simulink model "SPMe_EqCM"  (R2024a)
settings: Solver=FixedStepAuto  StartTime=0.0  StopTime=t_end  FixedStep=dt  MaxStep=1  RelTol=1e-6
values from neighbouring files (symbols this model uses):
  alpha = 64.526    [EqCM.m]
  dt = 0.2    [run_SPMe_fast_discharge.m]    (also in run_SPMe_sweep.m = param.dt; run_SPMe_vent.m = param.dt)
  I = 4.6*C_rates(c)    [run_SPMe_fast_discharge.m]    (also in run_SPMe_sweep.m; run_SPMe_vent.m = squeeze(sol.I.Data))
  p0 = [0.114319142120841  -0.663997904709863          1.686768366470837  -2.462409468590447   2.282769243949050          -1.401600551327618   0.576551904459066  -0.157044814050174          0.027351974716897  -0.002866912229499   0.000171009483610         0.000029999998915].*1e5    [run_SPMe_vent.m]
  Q_nom = 4.6    [run_SPMe_fast_discharge.m]    (also in run_SPMe_sweep.m; run_SPMe_vent.m)
  Rs = [0.051109270053841  -0.124390708105661             0.112323360710586  -0.046901650715843 0.015533047683140]             *z.^(4:-1:0)'    [EqCM.m]
  T_amb = 273.15+25    (= 298.15)    [EqCM.m]    (also in run_SPMe_vent.m = param.T_amb)
  V_min = 0    [run_SPMe_fast_discharge.m]    (also in run_SPMe_sweep.m; run_SPMe_vent.m = -3)
undefined symbols (not defined in the file or in its folder): A, DMC, E_p, EC, L_p0, m_an, M_C6, P_atm, P_crit, R, R_tab, sigma_0, SOC_0, V_head_0, x0, x_sei_0, y_dmc, y_ec
libraries: simulink x1
settings Model: Creator=tom  LastModifiedBy=Vivian
settings SolverCC: AlgebraicLoopSolver=TrustRegion
settings DebuggingCC: UnconnectedInputMsg=warning  UnconnectedOutputMsg=warning  UnconnectedLineMsg=warning
settings ModelReferenceCC: EnableRefExpFcnMdlSchedulingChecks=on
settings RTWCC: GPUComputeCapability=3.5  DLArmComputeVersion=19.05

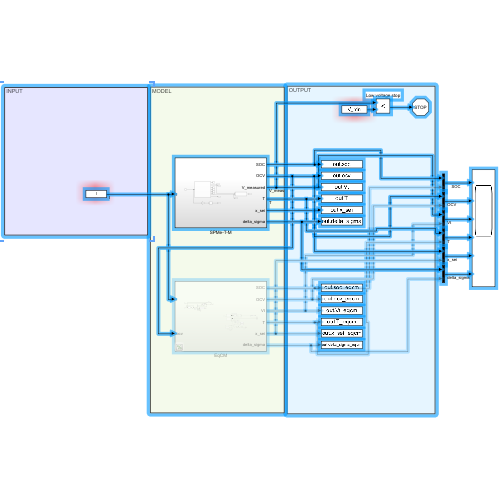
[thumbnail: Simulink's stored preview of the top-level diagram]
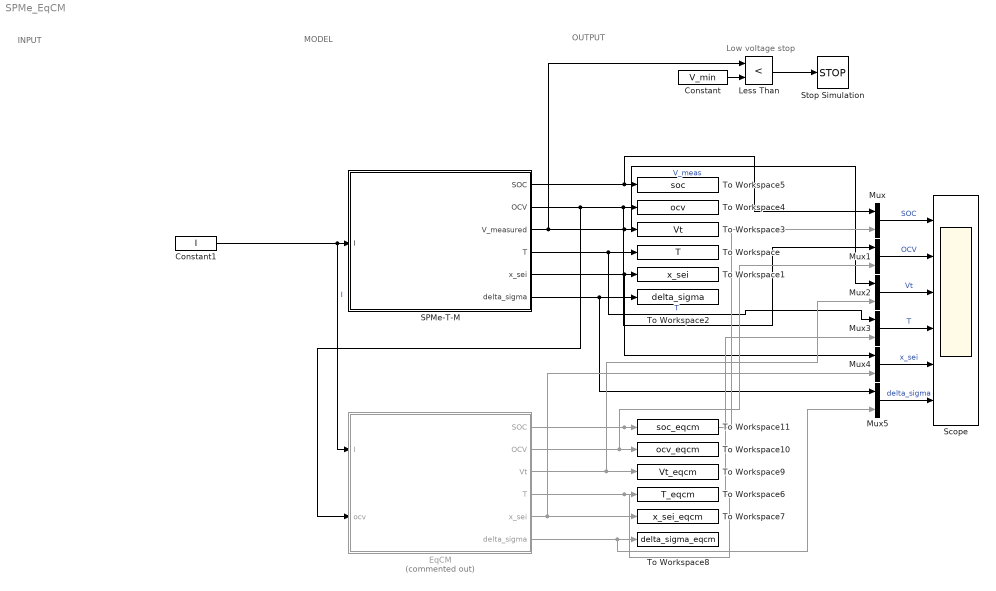
== system SPMe_EqCM ==
  note: OUTPUT
  note: MODEL
  note: INPUT
  note: Low voltage stop
  Constant : Constant  Value=V_min
  Constant1 : Constant  Value=I
  EqCM : Subsystem  Commented=on
  Less Than : RelationalOperator  Operator=<  OutDataTypeStr=boolean  RndMeth=Simplest  InputSameDT=off
  Mux{,1..5} (6 alike) : Mux  Inputs=2
  SPMe-T-M : Subsystem
  Scope : Scope  NumInputPorts=6
  Stop Simulation : Stop
  To Workspace : ToWorkspace  VariableName=T  SaveFormat=Timeseries  SampleTime=-1
  To Workspace1 : ToWorkspace  VariableName=x_sei  SaveFormat=Timeseries  SampleTime=-1
  To Workspace10 : ToWorkspace  VariableName=ocv_eqcm  SaveFormat=Timeseries  SampleTime=-1
  To Workspace11 : ToWorkspace  VariableName=soc_eqcm  SaveFormat=Timeseries  SampleTime=-1
  To Workspace2 : ToWorkspace  VariableName=delta_sigma  SaveFormat=Timeseries  SampleTime=-1
  To Workspace3 : ToWorkspace  VariableName=Vt  SaveFormat=Timeseries  SampleTime=-1
  To Workspace4 : ToWorkspace  VariableName=ocv  SaveFormat=Timeseries  SampleTime=-1
  To Workspace5 : ToWorkspace  VariableName=soc  SaveFormat=Timeseries  SampleTime=-1
  To Workspace6 : ToWorkspace  VariableName=T_eqcm  SaveFormat=Timeseries  SampleTime=-1
  To Workspace7 : ToWorkspace  VariableName=x_sei_eqcm  SaveFormat=Timeseries  SampleTime=-1
  To Workspace8 : ToWorkspace  VariableName=delta_sigma_eqcm  SaveFormat=Timeseries  SampleTime=-1
  To Workspace9 : ToWorkspace  VariableName=Vt_eqcm  SaveFormat=Timeseries  SampleTime=-1
  wires:
  Less Than/1 -> Stop Simulation/1
  Constant/1 -> Less Than/2
  SPMe-T-M/3(V_measured) -> Mux2/1, To Workspace3/1, Less Than/1  "V_meas"
  Constant1/1 -> EqCM/1(I), SPMe-T-M/1(I)  "I"
  SPMe-T-M/4(T) -> Mux3/1, To Workspace/1  "T"
  SPMe-T-M/5(x_sei) -> Mux4/1, To Workspace1/1
  SPMe-T-M/6(delta_sigma) -> Mux5/1, To Workspace2/1
  SPMe-T-M/2(OCV) -> EqCM/2(ocv), Mux1/1, To Workspace4/1
  SPMe-T-M/1(SOC) -> Mux/1, To Workspace5/1
  EqCM/1(SOC) -> Mux/2, To Workspace11/1
  EqCM/2(OCV) -> Mux1/2, To Workspace10/1
  EqCM/3(Vt) -> Mux2/2, To Workspace9/1
  EqCM/4(T) -> Mux3/2, To Workspace6/1
  Mux/1 -> Scope/1  "SOC"
  Mux1/1 -> Scope/2  "OCV"
  Mux2/1 -> Scope/3  "Vt"
  Mux3/1 -> Scope/4  "T"
  Mux4/1 -> Scope/5  "x_sei"
  Mux5/1 -> Scope/6  "delta_sigma"
  EqCM/5(x_sei) -> Mux4/2, To Workspace7/1
  EqCM/6(delta_sigma) -> Mux5/2, To Workspace8/1

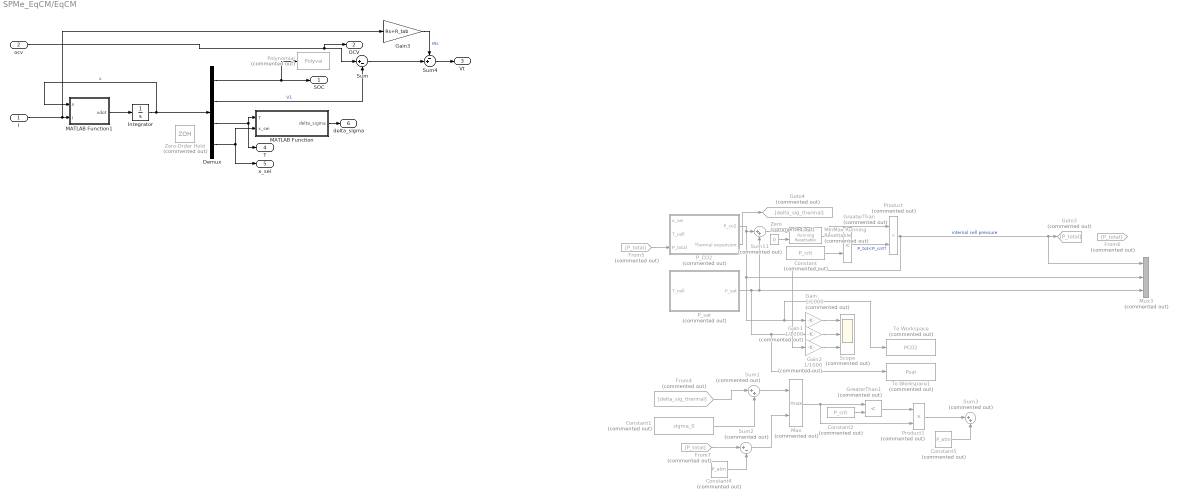
== system SPMe_EqCM/EqCM ==
  I : Inport
  ocv : Inport  Port=2
  Constant : Constant  Commented=on  Value=P_crit
  Constant1 : Constant  Commented=on  Value=sigma_0
  Constant2 : Constant  Commented=on  Value=P_crit
  Constant4 : Constant  Commented=on  Value=P_atm
  Constant5 : Constant  Commented=on  Value=P_atm
  Demux : Demux
  From4 : From  Commented=on  GotoTag=delta_sig_thermal
  From5 : From  Commented=on  GotoTag=P_total
  From6 : From  Commented=on  GotoTag=P_total
  From7 : From  Commented=on  GotoTag=P_total
  Gain : Gain  Commented=on  Gain=1/1000
  Gain1 : Gain  Commented=on  Gain=1/1000
  Gain2 : Gain  Commented=on  Gain=1/1000
  Gain3 : Gain  Gain=Rs+R_tab
  Goto3 : Goto  Commented=on  GotoTag=P_total
  Goto4 : Goto  Commented=on  GotoTag=delta_sig_thermal
  GreaterThan : RelationalOperator  Commented=on  Operator=<  OutDataTypeStr=boolean  RndMeth=Simplest  InputSameDT=off
  GreaterThan1 : RelationalOperator  Commented=on  Operator=<  OutDataTypeStr=boolean  RndMeth=Simplest  InputSameDT=off
  Integrator : Integrator  InitialCondition=x0'
  MATLAB Function : MATLAB Function  TreatAsAtomicUnit=on
  MATLAB Function1 : MATLAB Function  TreatAsAtomicUnit=on
  Max : MinMax  Commented=on  Function=max  Inputs=2
  MinMax Running Resettable : simulink/Math Operations/MinMax Running Resettable  Commented=on  Function=max  vinit=0
  Mux3 : Mux  Commented=on  Inputs=3
  P_CO2 : Subsystem  Commented=on
  P_sat : Subsystem  Commented=on
  Polynomial : Polyval  Commented=on  Coefs=p0
  Product : Product  Commented=on
  Product1 : Product  Commented=on
  Scope : Scope  Commented=on  NumInputPorts=3
  Sum : Sum  Inputs=|+-
  Sum1 : Sum  Commented=on  Inputs=|++
  Sum11 : Sum  Commented=on  Inputs=|++
  Sum2 : Sum  Commented=on  Inputs=|+-
  Sum3 : Sum  Commented=on  Inputs=|++
  Sum4 : Sum  Inputs=-+|
  To Workspace : ToWorkspace  Commented=on  VariableName=PCO2  SaveFormat=Timeseries  SampleTime=-1
  To Workspace1 : ToWorkspace  Commented=on  VariableName=Psat  SaveFormat=Timeseries  SampleTime=-1
  Zero : Constant  Commented=on  Value=0  OutDataTypeStr=Inherit: Inherit via back propagation
  Zero-Order Hold : ZeroOrderHold  Commented=on  SampleTime=dt
  SOC : Outport
  OCV : Outport  Port=2
  Vt : Outport  Port=3
  T : Outport  Port=4
  x_sei : Outport  Port=5
  delta_sigma : Outport  Port=6
  wires:
  I/1 -> Gain3/1, MATLAB Function1/2(I)
  From7/1 -> Sum2/1
  Sum11/1 -> MinMax Running Resettable/1
  Zero/1 -> MinMax Running Resettable/2
  GreaterThan/1 -> Product/2  "P_tot<P_crit?"
  Gain2/1 -> Scope/3
  Constant1/1 -> Sum1/2
  Constant4/1 -> Sum2/2
  Constant/1 -> GreaterThan/2
  Sum1/1 -> Max/1
  Constant2/1 -> GreaterThan1/2
  P_sat/1(P_sat) -> To Workspace1/1, Gain1/1, Sum11/2, Mux3/3
  Constant5/1 -> Sum3/2
  MinMax Running Resettable/1 -> Product/1, GreaterThan/1
  Product1/1 -> Sum3/1
  From4/1 -> Sum1/1
  Gain/1 -> Scope/1
  From5/1 -> P_CO2/3(P_total)
  Product/1 -> Gain2/1, Mux3/1, Goto3/1  "internal cell pressure"
  Max/1 -> GreaterThan1/1, Product1/2
  Gain1/1 -> Scope/2
  GreaterThan1/1 -> Product1/1
  P_CO2/1(P_co2) -> To Workspace/1, Gain/1, Mux3/2, Sum11/1
  P_CO2/2(Thermal expansion) -> Goto4/1
  Sum2/1 -> Max/2
  MATLAB Function/1(delta_sigma) -> delta_sigma/1
  MATLAB Function1/1(xdot) -> Integrator/1
  Integrator/1 -> Demux/1, MATLAB Function1/1(x)  "x"
  Demux/3 -> T/1, MATLAB Function/1(T)
  Demux/4 -> x_sei/1, MATLAB Function/2(x_sei)
  Demux/1 -> Polynomial/1, SOC/1
  Demux/2 -> Sum/2  "V1"
  Gain3/1 -> Sum4/1  "IRs"
  Sum/1 -> Sum4/2
  Sum4/1 -> Vt/1
  ocv/1 -> OCV/1, Sum/1

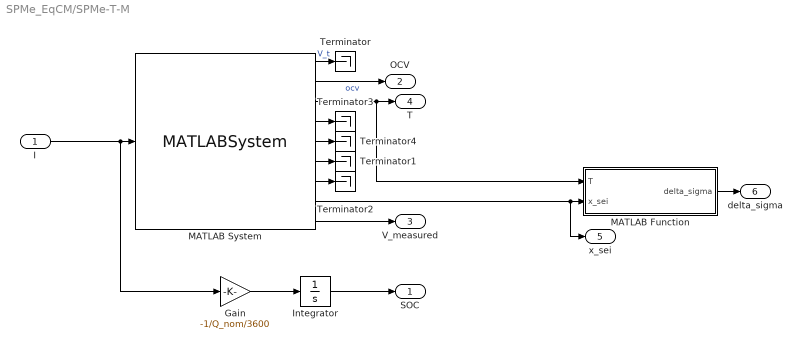
== system SPMe_EqCM/SPMe-T-M ==
  I : Inport
  Gain : Gain  Gain=-1/Q_nom/3600
  Integrator : Integrator  InitialCondition=SOC_0
  MATLAB Function : MATLAB Function  TreatAsAtomicUnit=on
  MATLAB System : MATLABSystem  System=pybamm_bat  SimulateUsing=Interpreted execution
      mask Type: pybamm_bat
      mask Display:
      | disp('pybamm_bat');
      | port_label('input',1,'current');
      | port_label('output',1,'V_t');
      | port_label('output',2,'ocv');
      | port_label('output',3,'T');
      | port_label('output',4,'ce');
      | port_label('output',5,'heating');
      | port_label('output',6,'neg_conc');
      | port_label('output',7,'pos_conc');
      | port_label('output',8,'x_sei');
      | port_label('output',9,'V_meas');
  Terminator{,1..4} (5 alike) : Terminator
  SOC : Outport
  OCV : Outport  Port=2
  V_measured : Outport  Port=3
  T : Outport  Port=4
  x_sei : Outport  Port=5
  delta_sigma : Outport  Port=6
  wires:
  MATLAB System/9 -> V_measured/1
  MATLAB System/3 -> MATLAB Function/1(T), T/1
  MATLAB System/8 -> x_sei/1, MATLAB Function/2(x_sei)
  MATLAB Function/1(delta_sigma) -> delta_sigma/1
  MATLAB System/1 -> Terminator/1  "V_t"
  MATLAB System/6 -> Terminator1/1
  MATLAB System/7 -> Terminator2/1
  MATLAB System/4 -> Terminator3/1
  MATLAB System/5 -> Terminator4/1
  MATLAB System/2 -> OCV/1  "ocv"
  I/1 -> Gain/1, MATLAB System/1
  Integrator/1 -> SOC/1
  Gain/1 -> Integrator/1

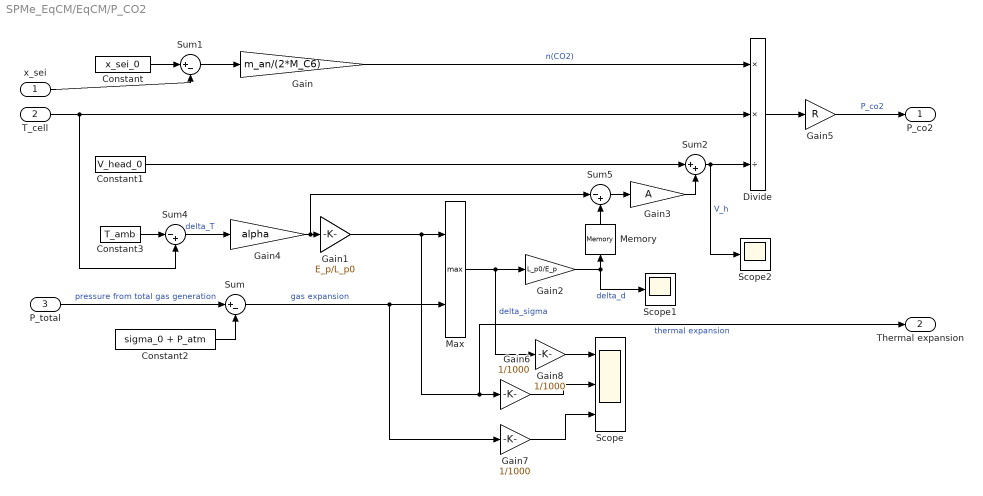
== system SPMe_EqCM/EqCM/P_CO2 ==
  x_sei : Inport
  T_cell : Inport  Port=2
  P_total : Inport  Port=3
  Constant : Constant  Value=x_sei_0
  Constant1 : Constant  Value=V_head_0
  Constant2 : Constant  Value=sigma_0 + P_atm
  Constant3 : Constant  Value=T_amb
  Divide : Product  Inputs=**/
  Gain : Gain  Gain=m_an/(2*M_C6)
  Gain1 : Gain  Gain=E_p/L_p0
  Gain2 : Gain  Gain=L_p0/E_p
  Gain3 : Gain  Gain=A
  Gain4 : Gain  Gain=alpha
  Gain5 : Gain  Gain=R
  Gain6 : Gain  Gain=1/1000
  Gain7 : Gain  Gain=1/1000
  Gain8 : Gain  Gain=1/1000
  Max : MinMax  Function=max  Inputs=2
  Memory : Memory
  Scope : Scope  NumInputPorts=3
  Scope1 : Scope
  Scope2 : Scope
  Sum : Sum  Inputs=|+-
  Sum1 : Sum  Inputs=|+-
  Sum2 : Sum  Inputs=|++
  Sum4 : Sum  Inputs=|-+
  Sum5 : Sum  Inputs=|-+
  P_co2 : Outport
  Thermal expansion : Outport  Port=2
  wires:
  Sum4/1 -> Gain4/1  "delta_T"
  Gain2/1 -> Scope1/1, Memory/1  "delta_d"
  Constant1/1 -> Sum2/1
  Sum1/1 -> Gain/1
  T_cell/1 -> Divide/2, Sum4/2
  Divide/1 -> Gain5/1
  Sum5/1 -> Gain3/1
  Max/1 -> Gain8/1, Gain2/1  "delta_sigma"
  Gain4/1 -> Sum5/1, Gain1/1
  Gain5/1 -> P_co2/1  "P_co2"
  Constant/1 -> Sum1/1
  Gain3/1 -> Sum2/2
  Gain/1 -> Divide/1  "n(CO2)"
  Sum2/1 -> Scope2/1, Divide/3  "V_h"
  Constant3/1 -> Sum4/1
  x_sei/1 -> Sum1/2
  Gain7/1 -> Scope/3
  Gain1/1 -> Thermal expansion/1, Gain6/1, Max/1  "thermal expansion"
  Memory/1 -> Sum5/2
  Sum/1 -> Gain7/1, Max/2  "gas expansion"
  P_total/1 -> Sum/1  "pressure from total gas generation"
  Constant2/1 -> Sum/2
  Gain6/1 -> Scope/2
  Gain8/1 -> Scope/1

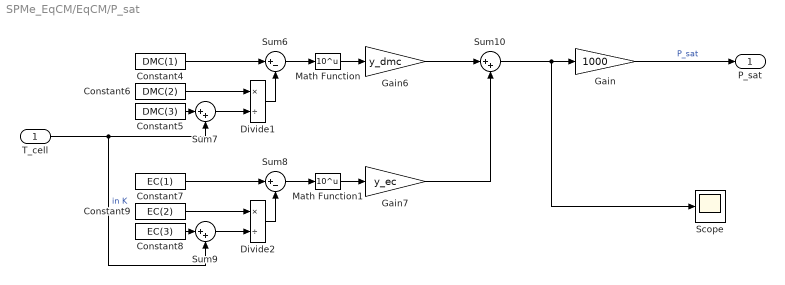
== system SPMe_EqCM/EqCM/P_sat ==
  T_cell : Inport
  Constant4 : Constant  Value=DMC(1)
  Constant5 : Constant  Value=DMC(3)
  Constant6 : Constant  Value=DMC(2)
  Constant7 : Constant  Value=EC(1)
  Constant8 : Constant  Value=EC(3)
  Constant9 : Constant  Value=EC(2)
  Divide1 : Product  Inputs=*/
  Divide2 : Product  Inputs=*/
  Gain : Gain  Gain=1000
  Gain6 : Gain  Gain=y_dmc
  Gain7 : Gain  Gain=y_ec
  Math Function : Math  Operator=10^u
  Math Function1 : Math  Operator=10^u
  Scope : Scope
  Sum10 : Sum  Inputs=|++
  Sum6 : Sum  Inputs=|+-
  Sum7 : Sum  Inputs=|++
  Sum8 : Sum  Inputs=|+-
  Sum9 : Sum  Inputs=|++
  P_sat : Outport
  wires:
  Constant7/1 -> Sum8/1
  Math Function1/1 -> Gain7/1
  Sum9/1 -> Divide2/2
  Sum6/1 -> Math Function/1
  Sum7/1 -> Divide1/2
  Divide2/1 -> Sum8/2
  T_cell/1 -> Sum9/2, Sum7/2  "in K"
  Constant4/1 -> Sum6/1
  Math Function/1 -> Gain6/1
  Constant8/1 -> Sum9/1
  Sum8/1 -> Math Function1/1
  Constant9/1 -> Divide2/1
  Divide1/1 -> Sum6/2
  Constant5/1 -> Sum7/1
  Constant6/1 -> Divide1/1
  Gain6/1 -> Sum10/1
  Gain7/1 -> Sum10/2
  Sum10/1 -> Scope/1, Gain/1
  Gain/1 -> P_sat/1  "P_sat"

== matlab function SPMe_EqCM/SPMe-T-M/MATLAB Function ==
  data: T input; x_sei input; delta_sigma output
function delta_sigma  = expansion(T,x_sei)
%XSEI2PTOTAL 
% Mechanical params
M_C6 = 72/1000; %kg/mol
% V_head_0 = 6.65e-6; %m3 (0.121*0.074*0.0055)*0.135
% L = 2.4/1000; %m
% E = 0.19e6; %Pa
% alpha_cell = 1.1e-6; %m/K
% P_atm = 101; %kPa
% P_crit = 158.7731; %kPa
R = 8.3145; %J.mol-1.K-1
A = 0.009; %m2 (0.121*0.074)
DMC = [6.4338; 1413; -44.25]; %Antoine coeffs [A B C] 
EC = [6.4897; 1836.57; -102.23];
y_dmc = 0.7;
y_ec = 1-y_dmc;         
m_an = 0.0191; 
x_sei_0 = 0.15;
% T_amb = 273.15+25; % K
% sigma_0 = 1.5120e+04;

% Internal cell pressure
V_head_0 = 6.65e-06; %m-3
L_p0 = 2.4e-3; %m for 2 poron
E_p = 0.19e6; %Pa Young's modulus for poron
% E_c = 1e12; %assume large by default
alpha = 1.1e-6; %m/K
P_atm = 101e3; %Pa
% P_crit = 158e3; %Pa
% P0 = 14e3; %Pa
R = 8.3145; %J.mol-1.K-1
% k_b = 1.380649e-23; %m2.kg.s-2.K-1;
T_amb = 273.15+25; % K
sigma_0 = 1.5120e+04;
% L_cs0 = 5.5e-3; %m initial cell solid thickness
% V_cell = 0.130*0.089*0.055; % [130mm×89mm×5.5mm] active material

% P_elyte
Psat_EC = 10.^(EC(1)-EC(2)./(EC(3)+T));
Psat_DMC = 10.^(DMC(1)-DMC(2)./(DMC(3)+T)); 
P_elyte = (y_dmc*Psat_DMC + y_ec*Psat_EC)*1e3; 

% P_CO2
n_CO2 = 0.5*m_an/M_C6*(x_sei_0-x_sei);

% Solve for gas volume and pressure
delta_sigma_calc = P_elyte - sigma_0 - P_atm;
a = 1;
b = -(V_head_0 + A.*(L_p0/E_p*(delta_sigma_calc) - alpha.*(T-T_amb)));
c = -A*L_p0/E_p.*n_CO2.*R.*(T);
V_g0 = (-b+sqrt(max(b.^2-4.*a.*c,0)))/(2*a);
V_g = max(V_g0, V_head_0); % min V_g = V_head_0

P_CO2 = n_CO2.*R.*T./V_g;
P_gas = P_elyte + P_CO2;

delta_sigma = max(P_gas-P_atm-sigma_0, E_p./L_p0.*alpha.*(T-T_amb));
end

== matlab function SPMe_EqCM/EqCM/MATLAB Function1 ==
  data: x input; xdot output; I input
function xdot = EqCM(x,I)
    z = x(1);
    V1 = x(2);
    T = x(3); 
    x_sei = x(4); 

    % ELECTRICAL 
    Q = 4.6; %A.h
    alpha = 1; %64.526;
    beta = 1; %; 0.48053;
    soc_ref=0.5; % remove SOC dependence
    Rs = [0.051109270053841  -0.124390708105661...
            0.112323360710586  -0.046901650715843 0.015533047683140]...
            *soc_ref.^(4:-1:0)';
    R1 = [0.030297671277692  -0.078249784854926...
        0.076106125220171  -0.035096138367922   0.013959006299232]...
        *soc_ref.^(4:-1:0)'*alpha;
    C1 = [-0.178332712122388   0.724802617995660 ...
        -1.060271845888578   0.759649001977427   0.210118417436246]...
        *1e4*soc_ref.^(4:-1:0)'*beta;
    
    S = diag([0 -1/(R1*C1)]);
    xdot_e = S*[z V1]' + [-1/Q/3600 1/C1]'*I; 



    % SEI DECOMPOSITION
    A_sei = 2.25e15*0.13210066; %s-1
    E_sei = 2.24e-19; %J
    k_b = 1.3806e-23; %J.K-1
%     x_sei_0 = 0.15; %initial fraction of Li in SEI
    x_sei_dot = -A_sei*exp(-E_sei/k_b/T)*x_sei;


    % THERMAL
    hA = 0.4865;
    mCp =  219.2578;
    T_amb = 273.15+25; % K
    m_an = 0.0191;
    h_sei =257000;
    Q_sei = m_an*h_sei*x_sei_dot;
    R_tab = 0086;
    Tdot = 1/mCp*(I*(V1+Rs*I) + Q_sei)- hA/mCp*(T-T_amb); %redefine deltaV?
   
    % Recombine states
	xdot = [xdot_e;Tdot;x_sei_dot];
end

== matlab function SPMe_EqCM/EqCM/MATLAB Function ==
  data: T input; x_sei input; delta_sigma output
function delta_sigma  = expansion(T,x_sei)
%XSEI2PTOTAL 
% Mechanical params
M_C6 = 72/1000; %kg/mol
% V_head_0 = 6.65e-6; %m3 (0.121*0.074*0.0055)*0.135
% L = 2.4/1000; %m
% E = 0.19e6; %Pa
% alpha_cell = 1.1e-6; %m/K
% P_atm = 101; %kPa
% P_crit = 158.7731; %kPa
R = 8.3145; %J.mol-1.K-1
A = 0.009; %m2 (0.121*0.074)
DMC = [6.4338; 1413; -44.25]; %Antoine coeffs [A B C] 
EC = [6.4897; 1836.57; -102.23];
y_dmc = 0.7;
y_ec = 1-y_dmc;         
m_an = 0.0191; 
x_sei_0 = 0.15;
% T_amb = 273.15+25; % K
% sigma_0 = 1.5120e+04;

% Internal cell pressure
V_head_0 = 6.65e-06; %m-3
L_p0 = 2.4e-3; %m for 2 poron
E_p = 0.19e6; %Pa Young's modulus for poron
% E_c = 1e12; %assume large by default
alpha = 1.1e-6; %m/K
P_atm = 101e3; %Pa
% P_crit = 158e3; %Pa
% P0 = 14e3; %Pa
R = 8.3145; %J.mol-1.K-1
% k_b = 1.380649e-23; %m2.kg.s-2.K-1;
T_amb = 273.15+25; % K
sigma_0 = 1.5120e+04;
% L_cs0 = 5.5e-3; %m initial cell solid thickness
% V_cell = 0.130*0.089*0.055; % [130mm×89mm×5.5mm] active material

% P_elyte
Psat_EC = 10.^(EC(1)-EC(2)./(EC(3)+T));
Psat_DMC = 10.^(DMC(1)-DMC(2)./(DMC(3)+T)); 
P_elyte = (y_dmc*Psat_DMC + y_ec*Psat_EC)*1e3; 

% P_CO2
n_CO2 = 0.5*m_an/M_C6*(x_sei_0-x_sei);

% Solve for gas volume and pressure
delta_sigma_calc = P_elyte - sigma_0 - P_atm;
a = 1;
b = -(V_head_0 + A.*(L_p0/E_p*(delta_sigma_calc) - alpha.*(T-T_amb)));
c = -A*L_p0/E_p.*n_CO2.*R.*(T);
V_g0 = (-b+sqrt(max(b.^2-4.*a.*c,0)))/(2*a);
V_g = max(V_g0, V_head_0); % min V_g = V_head_0

P_CO2 = n_CO2.*R.*T./V_g;
P_gas = P_elyte + P_CO2;

delta_sigma = max(P_gas-P_atm-sigma_0, E_p./L_p0.*alpha.*(T-T_amb));
end
